simulink library "CtrlSurfMapping_Lib"  (Simulink 8.0)
settings: Solver=ode45  StartTime=0.0  StopTime=10.0  RelTol=1e-3
undefined symbols (not defined in the file): AC
libraries: CtrlSurfMapping_Lib x1
settings Model: Creator=hpfifer  LastModifiedBy=brtaylor

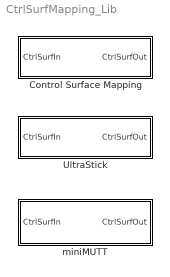
== system CtrlSurfMapping_Lib ==
  Control Surface Mapping : Subsystem  BlockChoice=UltraStick  mask{aircraft=AC.aircraft}
      mask prompts: aircraft "Aircraft type:"
      mask init:
      | pathname = gcb;
      | 
      | switch lower(aircraft)
      |     case 'ultrastick120'
      |         set_param(pathname,'BlockChoice','UltraStick');
      |    case 'ultrastick25e'
      |         set_param(pathname,'BlockChoice','UltraStick');
      |     case 'minimutt'
      |         set_param(pathname,'BlockChoice','miniMUTT');
      | end
      settings: TemplateBlock=self  MemberBlocks=UltraStick,miniMUTT
  UltraStick : Subsystem
  miniMUTT : Subsystem

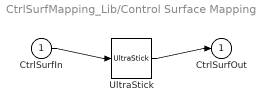
== system CtrlSurfMapping_Lib/Control Surface Mapping ==
  CtrlSurfIn : Inport
  UltraStick : CtrlSurfMapping_Lib/UltraStick
  CtrlSurfOut : Outport
  wires:
  CtrlSurfIn/1 -> UltraStick/1
  UltraStick/1 -> CtrlSurfOut/1

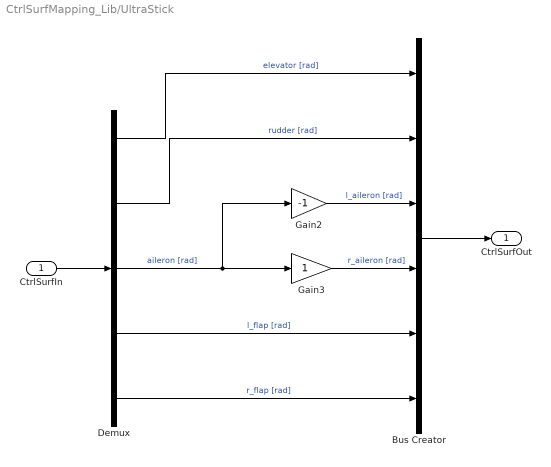
== system CtrlSurfMapping_Lib/UltraStick ==
  CtrlSurfIn : Inport
  Bus Creator : BusCreator  Inputs=6
  Demux : Demux  Outputs=5
  Gain2 : Gain  Gain=-1
  Gain3 : Gain
  CtrlSurfOut : Outport
  wires:
  CtrlSurfIn/1 -> Demux/1
  Bus Creator/1 -> CtrlSurfOut/1
  Demux/3 -> Gain2/1, Gain3/1  "aileron [rad]"
  Gain2/1 -> Bus Creator/3  "l_aileron [rad]"
  Gain3/1 -> Bus Creator/4  "r_aileron [rad]"
  Demux/1 -> Bus Creator/1  "elevator [rad]"
  Demux/4 -> Bus Creator/5  "l_flap [rad]"
  Demux/5 -> Bus Creator/6  "r_flap [rad]"
  Demux/2 -> Bus Creator/2  "rudder [rad]"

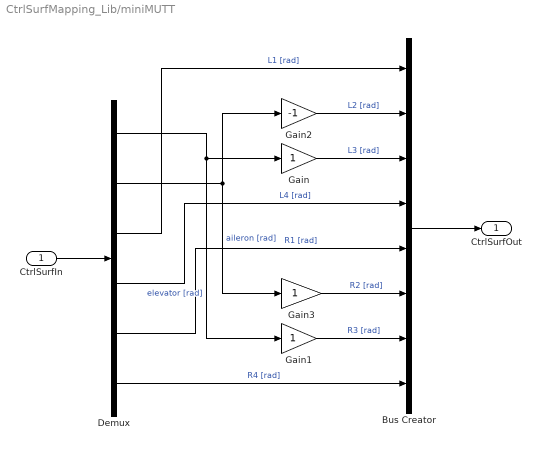
== system CtrlSurfMapping_Lib/miniMUTT ==
  CtrlSurfIn : Inport
  Bus Creator : BusCreator  Inputs=8
  Demux : Demux  Outputs=6
  Gain : Gain
  Gain1 : Gain
  Gain2 : Gain  Gain=-1
  Gain3 : Gain
  CtrlSurfOut : Outport
  wires:
  CtrlSurfIn/1 -> Demux/1
  Bus Creator/1 -> CtrlSurfOut/1
  Demux/1 -> Gain/1, Gain1/1  "elevator [rad]"
  Gain/1 -> Bus Creator/3  "L3 [rad]"
  Gain1/1 -> Bus Creator/7  "R3 [rad]"
  Demux/2 -> Gain3/1, Gain2/1  "aileron [rad]"
  Gain2/1 -> Bus Creator/2  "L2 [rad]"
  Gain3/1 -> Bus Creator/6  "R2 [rad]"
  Demux/3 -> Bus Creator/1  "L1 [rad]"
  Demux/4 -> Bus Creator/4  "L4 [rad]"
  Demux/5 -> Bus Creator/5  "R1 [rad]"
  Demux/6 -> Bus Creator/8  "R4 [rad]"
